simulink model "demo_FIXS"  (R2024a)
settings: Solver=VariableStepAuto  StartTime=0.0  StopTime=10.0  RelTol=1e-3
PostLoadFcn:
  | if any(exist('dsrtsu_mdlpostloadfcn', 'file') ~= 0), dsrtsu_mdlpostloadfcn('Execute', bdroot); end
InitFcn:
  | , if any(exist('dsmpb_private', 'file') ~= 0), dsmpb_private('dsmpb_mdlclblib', 'Init', bdroot); end,
values from neighbouring files (symbols this model uses):
  RealSimPara =     [Run_Simulink.mat]
libraries: dsmpblib x7, simulink x2
PreSaveFcn:
  | , if any(exist('dsmpb_private', 'file') ~= 0), dsmpb_private('dsmpb_mdlclblib', 'PreSave', bdroot); end,
CloseFcn:
  | , if any(exist('dsmpb_private', 'file') ~= 0), dsmpb_private('dsmpb_mdlclblib', 'Close', bdroot); end,
settings Model: DSMPB_ID_DATA={'114',struct('BlockId','a362e819-36dc-4974-aa36-3021815529a3','SignalIds',{{'66e99ec9-adbb-4575-a499-7c125ba92483'}}),'126',struct('BlockId','ae842df5-44fe-466f-9c27-a215b2028e86','SignalIds',{{'c9fc9f6b-9f86-4efb-bbc4-57bab20bb633'}}),'127',struct('BlockId','bbe675d0-07e1-4678-85bf-fdbba0576f1e','SignalIds',{{'fbad8ef8-ed8e-4d52-83c5-289887b658bf','bfa4259a-ff07-4a65-a7c9-9af4643f0ea5','da3d735e-2e4d-4dbe-9156-097bd40e1eb5','0aaec2e5-1bc6-40e3-804f-bcf62d1171e8'}}),'128',struct('BlockId','76c42765-af6a-43b1-a646-d573c8b7c57f','SignalIds',{{'afa686ea-bff9-4ae8-bbc4-1f85da76ddbd'}}),'129',struct('BlockId','547cde89-fa54-43bb-91af-f85d56e956d9','SignalIds',{{'71dcf01e-4040-4f0f-9727-35b21fbf9010'}}),'134',struct('BlockId','2d3928d4-db37-4811-a604-a01aef7cb2d7','SignalIds',{{'b231ed0e-9922-4662-b18e-0578afdeacb1','d97ae3f2-e654-4125-b1b8-791beb64344e'}}),'147',struct('BlockId','e4d38646-31b4-470f-bd5f-0342a996991a','SignalIds',{{'19e5aa06-a56a-40dc-84e8-1ac500eeaf07','77e1adf7-a3b1-4325-a85b-daf2ff9418b5','6e5fcfab-5f3b-494e-8d3b-0a2c9e0cd453'}})}  Creator=MSC_Lab  LastModifiedBy=MSC_Lab

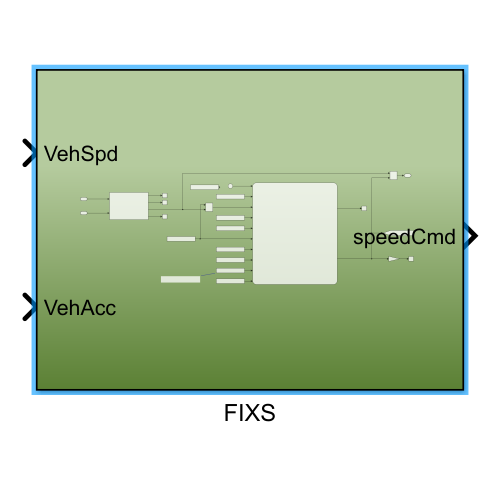
[thumbnail: Simulink's stored preview of the top-level diagram]
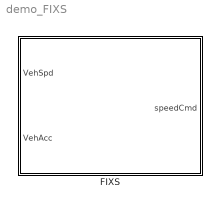
== system demo_FIXS ==
  FIXS : Subsystem

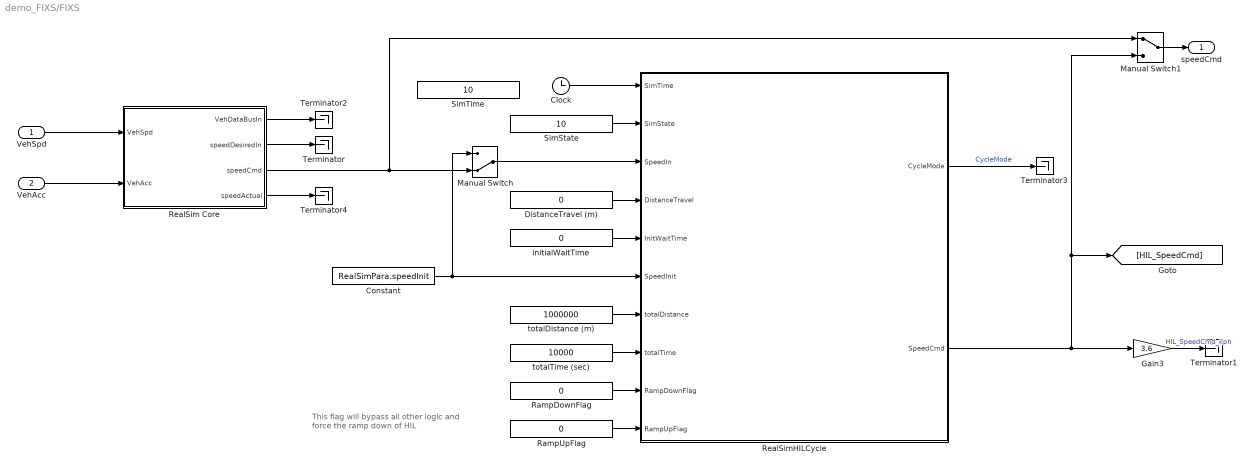
== system demo_FIXS/FIXS ==
  note: This flag will bypass all other logic and force the ramp down of HIL
  VehSpd : Inport
  VehAcc : Inport  Port=2
  Clock : Clock
  Constant : Constant  Value=RealSimPara.speedInit
  DistanceTravel (m) : Constant  Value=0
  Gain3 : Gain  Gain=3.6
  Manual Switch : ManualSwitch  CurrentSetting=0
  Manual Switch1 : ManualSwitch
  RampDownFlag : Constant  Value=0
  RampUpFlag : Constant  Value=0
  RealSim Core : Subsystem
  RealSimHILCycle : Stateflow chart  TreatAsAtomicUnit=on
  SimState : Constant  Value=10
  SimTime : Constant  Value=10
  Terminator{,1..4} (5 alike) : Terminator
  initialWaitTime : Constant  Value=0
  totalDistance (m) : Constant  Value=1000000
  totalTime (sec) : Constant  Value=10000
  speedCmd : Outport
  wires:
  RealSim Core/2(speedDesiredIn) -> Terminator/1
  RampDownFlag/1 -> RealSimHILCycle/9(RampDownFlag)
  totalDistance (m)/1 -> RealSimHILCycle/7(totalDistance)
  Manual Switch/1 -> RealSimHILCycle/3(SpeedIn)
  Gain3/1 -> Terminator1/1  "HIL_SpeedCmd_kph"
  totalTime (sec)/1 -> RealSimHILCycle/8(totalTime)
  RealSimHILCycle/1(CycleMode) -> Terminator3/1  "CycleMode"
  initialWaitTime/1 -> RealSimHILCycle/5(InitWaitTime)
  RealSimHILCycle/2(SpeedCmd) -> [HIL_SpeedCmd], Manual Switch1/2, Gain3/1
  Constant/1 -> Manual Switch/1, RealSimHILCycle/6(SpeedInit)
  Manual Switch1/1 -> speedCmd/1
  RealSim Core/3(speedCmd) -> Manual Switch1/1, Manual Switch/2
  RampUpFlag/1 -> RealSimHILCycle/10(RampUpFlag)
  VehSpd/1 -> RealSim Core/1(VehSpd)
  RealSim Core/1(VehDataBusIn) -> Terminator2/1
  RealSim Core/4(speedActual) -> Terminator4/1
  DistanceTravel (m)/1 -> RealSimHILCycle/4(DistanceTravel)
  SimState/1 -> RealSimHILCycle/2(SimState)
  Clock/1 -> RealSimHILCycle/1(SimTime)
  VehAcc/1 -> RealSim Core/2(VehAcc)

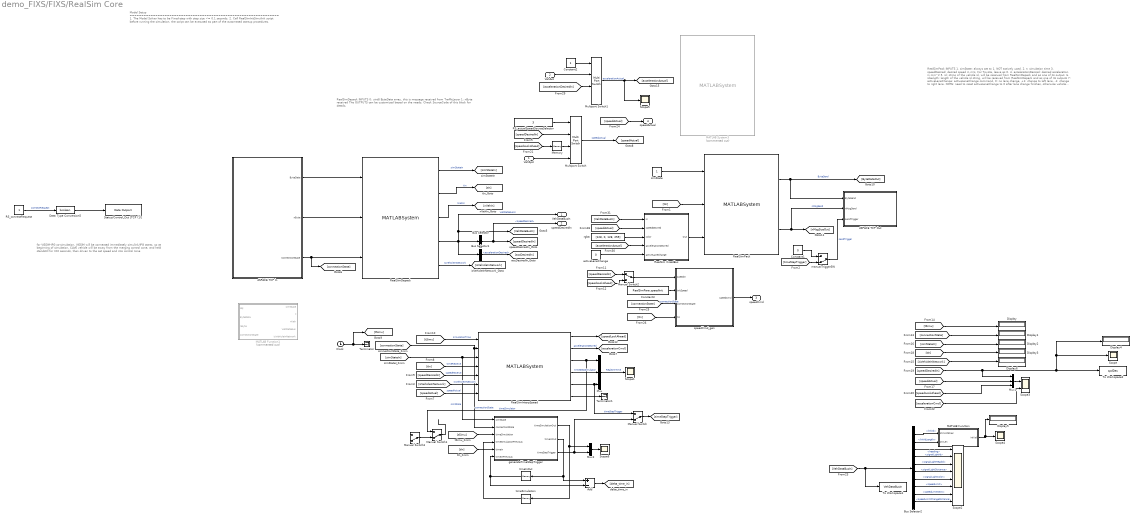
== system demo_FIXS/FIXS/RealSim Core ==
  note: Model Setup
      | ================================================================
      | 1. The Model Solver has to be Fixed-step with step size <= 0.1 seconds.
      | 2. Call RealSimInitSimulink script before running the simulation. the script can be executed as part of the automated startup procedures.
  note: RealSimDepack
      | INPUTS
      | 0: uint8 ByteData array, this is message received from TrafficLayer
      | 1: nByte received
      |
      | The OUTPUTS can be customized based on the needs. Check SourceCode of this block for details.
  note: RealSimPack
      | INPUTS
      | 1. simState: always set to 1. NOT actively used.
      | 2. t: simulation time
      | 3. speedDesired: desired speed in m/s, For Toyota, leave as 0.
      | 4. accelerationDesired: desired acceleration in m/s^2
      | 5. id: string of the vehicle id, will be received from RealSimDepack and as one of its output.
      | 6. idLength: length of the vehicle id string, will be received from RealSimDepack and as one of its outputs
      | 7: activeLaneChange: activeLaneChange command, 0: no lane change, +1: change to left lane, -1: change to right lane. NOTE: need to reset activeLaneChange to 0 after lane change finishes, otherwise vehicle will keep making lane change. Will receive 0 activeLaneChangeFdbk from RealSimDepack when lane change finishes.
      |
      | NOTE 1: Currently, only speedDesired and/or accelerationDesired can be sent to VISSIM/SUMO. The data format receive and send are the same so other mesage fields of the send data are irrelevant and can be set to empty or zero.
      |
      | NOTE 2: if select both speedDesired and accelerationDesired
      | in config.yaml, then only accelerationDesired will be used
      | to control vehicles in TrafficSimulator. if only one of
      | speedDesired and accelerationDesired selected in
      | config.yaml, then the one selected will be used for
      | control, the other input can be leave as 0.
      |
      | NOTE 3: for VISSIM, speedDesired or accelerationDesired will be the control command 0.2 seconds in the future.
      |
      | OUTPUTS
      | 1.ByteData: bytes vector that will be sent to TrafficSimualtor
      | 2.nMsgSize: size of bytes to be sent
  note: for VISSIM-IPG co-simulation, VISSIM will be connected immediately simulink/IPG starts. so at beginning of simulation, CAVE vehicle will be away from the merging control zone, and held standstill for XXX seconds, then driven to the set speed and into control zone
  VehSpd : Inport
  VehAcc : Inport  Port=2
  Add : Sum  Inputs=+-
  Bus Selector : BusSelector  OutputSignals=speedDesired
  Bus Selector1 : BusSelector  OutputSignals=accelerationDesired
  Bus Selector2 : BusSelector  OutputSignals=linkId,linkIdLength,heading,signalLightId,signalLightHeadId,signalLightDistance,signalLightColor,speedLimit,speedLimitNext,speedLimitChangeDistance
  Clock : Clock
  Constant1 : Constant  Value=0
  Constant2 : Constant
  Constant3 : Constant  Value=RealSimPara.speedInit
  Data Type Conversion5 : DataTypeConversion  OutDataTypeStr=boolean  SaturateOnIntegerOverflow=off  RndMeth=Floor
  Display{,1..6} (7 alike) : Display
  MATLAB Function : MATLAB Function  TreatAsAtomicUnit=on
  MATLAB Function1 : MATLAB Function  Commented=on  TreatAsAtomicUnit=on
  MATLAB System3 : MATLABSystem  Commented=on  System=RealSimPack  VehicleMessageFieldDefInputVec=VehicleMessageFieldDefInputVec  SimulateUsing=Code generation
      mask Type: RealSimPack
      mask Display:
      | disp('RealSimPack');
      | port_label('input',1,'simState');
      | port_label('input',2,'t');
      | port_label('input',3,'VehDataBus');
      | port_label('output',1,'ByteData');
      | port_label('output',2,'nMsgSize');
  Manual Switch : ManualSwitch  CurrentSetting=0
  Manual Switch1 : ManualSwitch  CurrentSetting=0
  Manual Switch2 : ManualSwitch
  Manual Switch3 : ManualSwitch  CurrentSetting=0
  Memory : Memory
  Multiport Switch : MultiPortSwitch  SaturateOnIntegerOverflow=off  InputSameDT=off
  Multiport Switch1 : MultiPortSwitch  SaturateOnIntegerOverflow=off  InputSameDT=off
  Mux : Mux  Inputs=3
  Mux1 : Mux  Inputs=3
  Mux2 : Mux  Inputs=2
  RS_actualSpeedSourceSelector : Constant  Value=3
  RS_connectRequest : Constant
  RealSim CreatBus : Subsystem
  RealSimDepack : MATLABSystem  System=RealSimDepack  OutputBusName=VehDataBus  VehicleMessageFieldDefInputVec=VehicleMessageFieldDefInputVec  SimulateUsing=Code generation
      mask Type: RealSimDepack
      mask Display:
      | disp('RealSimDepack');
      | port_label('input',1,'ByteData');
      | port_label('input',2,'nByte');
      | port_label('input',3,'connectionState');
      | port_label('output',1,'simState');
      | port_label('output',2,'t');
      | port_label('output',3,'nVeh');
      | port_label('output',4,'VehDataBus');
      | port_label('output',5,'isVehicleInNetwork');
  RealSimInterpSpeed : MATLABSystem  System=RealSimInterpSpeed  initialSpeed=RealSimPara.speedInit  speedLookAheadHorizon=RealSimPara.tLookahead  speedUpperBound=30  smoothWindow=RealSimPara.smoothWindow  SimulateUsing=Code generation
      mask Type: RealSimInterpSpeed
      mask Display:
      | disp('RealSimInterpSpeed');
      | port_label('input',1,'simulationTime');
      | port_label('input',2,'connectionState');
      | port_label('input',3,'simState');
      | port_label('input',4,'timeReceive');
      | port_label('input',5,'speedReceive');
      | port_label('input',6,'isVehicleInNetwork');
      | port_label('input',7,'speedActual');
      | port_label('output',1,'speedLookAhead');
      | port_label('output',2,'accelerationDesired');
      | port_label('output',3,'timeSimulator');
      | port_label('output',4,'timeStepSimulator');
      | port_label('output',5,'timeStepTrigger');
      | port_label('output',6,'RealSimDelay');
  RealSimPack : MATLABSystem  System=RealSimPack  VehicleMessageFieldDefInputVec=VehicleMessageFieldDefInputVec  SimulateUsing=Code generation
      mask Type: RealSimPack
      mask Display:
      | disp('RealSimPack');
      | port_label('input',1,'simState');
      | port_label('input',2,'t');
      | port_label('input',3,'VehDataBus');
      | port_label('output',1,'ByteData');
      | port_label('output',2,'nMsgSize');
  Scope{,1,4..6} (5 alike) : Scope
  Scope2 : Scope  NumInputPorts=8
  Scope3 : Scope  NumInputPorts=2
  Status/Control_Out [TCP (1)] : dsmpblib/Data Outport  Priority=-10000
      settings: SourceProductName=dSPACE Model Interface Package for Simulink (MIPS)
  Terminator : Terminator
  Terminator1 : Terminator
  To Workspace1 : ToWorkspace  VariableName=VehDataBusIn  SaveFormat=Timeseries  SampleTime=-1
  To Workspace2 : ToWorkspace  VariableName=spdDes  SaveFormat=Structure With Time  SampleTime=-1
  activeLaneChange : Constant  Value=0
  dSPACE TCP In : Subsystem
  dSPACE TCP Out : Subsystem
  generateTimeStepTrigger : MATLAB Function  TreatAsAtomicUnit=on
  manualTriggerSW : ManualSwitch  CurrentSetting=0
  rgba : Constant  Value=[128, 0, 128, 255]
  simState : Constant
  speedCmd_gen : Subsystem
  timeInOut : Memory
  timeSimulation : Memory
  VehDataBusIn : Outport
  speedDesiredIn : Outport  Port=2
  speedCmd : Outport  Port=3
  speedActual : Outport  Port=4
  wires:
  [speedLookAhead] -> Memory/1
  Bus Selector/1 -> speedDesiredIn/1, [speedDesiredIn]  "<speedDesired>"
  RealSimDepack/1 -> [simStateIn]  "simStateIn"
  Bus Selector2/9 -> Scope2/7  "<speedLimitNext>"
  [tSimu] -> RealSimInterpSpeed/1  "simulationTime"
  RealSimInterpSpeed/4 -> Mux/2  "timeStepSimulator"
  Bus Selector2/1 -> MATLAB Function/1(strUint8Vec)  "<linkId>"
  Bus Selector2/3 -> Scope2/1  "<heading>"
  [tIn] -> RealSimInterpSpeed/4  "timeReceive"
  Bus Selector2/10 -> Scope2/8  "<speedLimitChangeDistance>"
  VehSpd/1 -> Multiport Switch/4
  [speedDesiredIn] -> RealSimInterpSpeed/5  "speedReceive"
  [simStateIn] -> Display2/1
  RealSimDepack/3 -> [nVehIn]  "nVehIn"
  [VehDataBusIn] -> To Workspace1/1, Bus Selector2/1
  [isVehicleInNetwork] -> Display6/1
  Bus Selector2/7 -> Scope2/5  "<signalLightColor>"
  simState/1 -> RealSimPack/1
  RealSimDepack/4 -> Bus Selector1/1, VehDataBusIn/1, [VehDataBusIn], Bus Selector/1  "VehDataBusIn"
  [speedDesiredIn] -> Display4/1, Scope/1, To Workspace2/1, Mux1/1
  RealSimInterpSpeed/2 -> [accelerationCmd]  "accelerationDesired"
  [isVehicleInNetwork] -> RealSimInterpSpeed/6  "isVehicleInNetwork"
  RS_actualSpeedSourceSelector/1 -> Multiport Switch/1
  RealSim CreatBus/1(Out) -> RealSimPack/3
  [accelerationCmd] -> Scope3/2
  Mux/1 -> Scope1/1  "RealSimTime"
  [tIn] -> RealSimPack/2
  Bus Selector2/2 -> MATLAB Function/2(strLen)  "<linkIdLength>"
  Bus Selector2/8 -> Scope2/6  "<speedLimit>"
  [connectionState] -> Display1/1
  RealSimInterpSpeed/5 -> Manual Switch/1, Mux/3  "timeStepTrigger"
  RealSimDepack/5 -> [isVehicleInNetwork]  "isVehicleInNetwork"
  Bus Selector2/5 -> Scope2/3  "<signalLightHeadId>"
  Bus Selector2/6 -> Scope2/4  "<signalLightDistance>"
  RealSimInterpSpeed/6 -> Terminator1/1
  RealSimPack/1 -> dSPACE TCP Out/1(ByteSend), [ByteDataOut]  "ByteSend"
  [tIn] -> Display3/1
  Multiport Switch/1 -> [speedActual]  "speedActual"
  [tSimu] -> Display/1
  [connectionState] -> generateTimeStepTrigger/2(connectionState), RealSimInterpSpeed/2  "connectionState"
  [speedLookAhead] -> Mux1/3
  [speedActual] -> RealSimInterpSpeed/7  "speedActual"
  [simStateIn] -> generateTimeStepTrigger/1(simState), RealSimInterpSpeed/3  "simState"
  RealSimInterpSpeed/1 -> [speedLookAhead]
  Mux1/1 -> Scope3/1
  MATLAB Function/1(intVal) -> Display5/1, Scope4/1
  RealSimPack/2 -> dSPACE TCP Out/2(nMsgSend), [nMsgSizeOut]  "nMsgSend"
  Bus Selector2/4 -> Scope2/2  "<signalLightId>"
  RealSimInterpSpeed/3 -> Mux/1, Manual Switch1/1  "timeSimulator"
  [speedDesiredIn] -> Multiport Switch/2
  [speedActual] -> Mux1/2
  RealSimDepack/2 -> [tIn]  "tIn"
  manualTriggerSW/1 -> dSPACE TCP Out/3(sendTrigger)  "sendTrigger"
  dSPACE TCP In/3(ConnectionState) -> RealSimDepack/3, [connectionState]
  dSPACE TCP In/1(ByteData) -> RealSimDepack/1
  dSPACE TCP In/2(nByte) -> RealSimDepack/2
  Data Type Conversion5/1 -> Status/Control_Out [TCP (1)]/1
  RS_connectRequest/1 -> Data Type Conversion5/1  "connectRequest"
  Memory/1 -> Multiport Switch/3
  Clock/1 -> Terminator/1, [tSimu]
  timeSimulation/1 -> generateTimeStepTrigger/4(timeSimulationPrevious)
  generateTimeStepTrigger/3(timeStepTrigger) -> Manual Switch/2, Mux2/2
  generateTimeStepTrigger/1(timeSimulationOut) -> Mux2/1, timeSimulation/1
  Mux2/1 -> Scope6/1
  Manual Switch/1 -> [timeStepTrigger]
  [timeStepTrigger] -> manualTriggerSW/2
  Constant1/1 -> manualTriggerSW/1
  ? -> Manual Switch3/1
  [speedDesiredIn] -> Manual Switch2/1
  [speedLookAhead] -> Manual Switch2/2
  [speedActual] -> speedActual/1
  Manual Switch2/1 -> speedCmd_gen/1(speedIn)
  Constant3/1 -> speedCmd_gen/2(initSpeed)
  speedCmd_gen/1(speedCmd) -> speedCmd/1
  [connectionState] -> speedCmd_gen/3(connectionState)  "connectionState"
  [tIn] -> speedCmd_gen/4(tIn)
  ? -> Manual Switch3/2
  Manual Switch3/1 -> Manual Switch1/2
  generateTimeStepTrigger/2(timeInOut) -> Add/1, timeInOut/1
  timeInOut/1 -> Add/2, generateTimeStepTrigger/6(timeInPrevious)
  [VehDataBusIn] -> RealSim CreatBus/1(In)
  rgba/1 -> RealSim CreatBus/3(color)
  activeLaneChange/1 -> RealSim CreatBus/5(activeLaneChange)
  [speedActual] -> RealSim CreatBus/2(speedDesired)
  Bus Selector1/1 -> [accDesiredIn]  "<accelerationDesired>"
  [accelerationDesiredIn] -> Multiport Switch1/3
  VehAcc/1 -> Multiport Switch1/2
  Constant2/1 -> Multiport Switch1/1
  Multiport Switch1/1 -> [accelerationActual], Scope5/1  "accelerationActual"
  [accelerationActual] -> RealSim CreatBus/4(accelerationDesired)
  Manual Switch1/1 -> ?
  [tSimu] -> generateTimeStepTrigger/3(timeSimulation)
  [tIn] -> generateTimeStepTrigger/5(timeIn)
  Add/1 -> [delta_time_in]

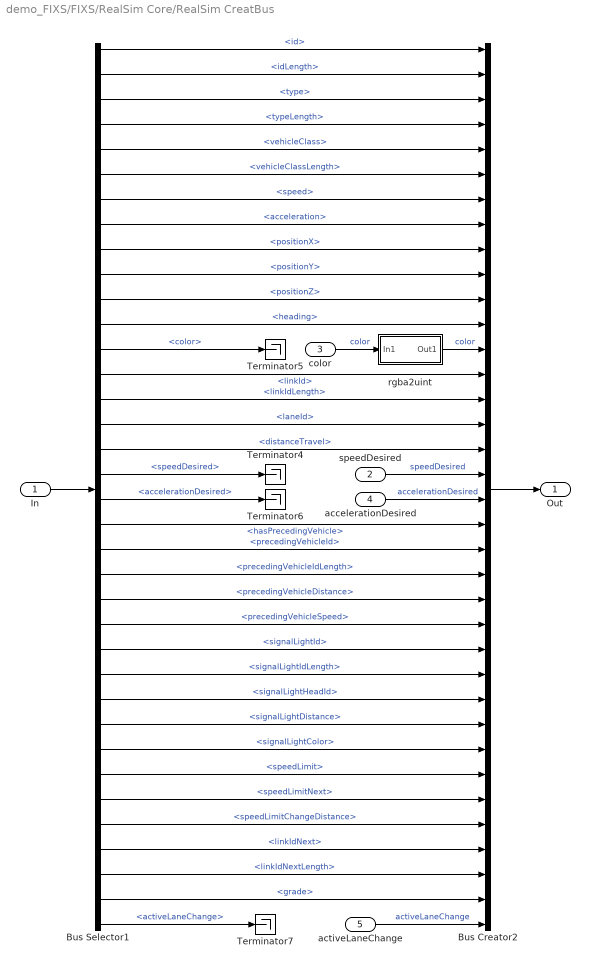
== system demo_FIXS/FIXS/RealSim Core/RealSim CreatBus ==
  In : Inport
  speedDesired : Inport  Port=2
  color : Inport  Port=3
  accelerationDesired : Inport  Port=4
  activeLaneChange : Inport  Port=5
  Bus Creator2 : BusCreator  Inputs=36  OutDataTypeStr=Bus: VehDataBus
  Bus Selector1 : BusSelector  OutputSignals=id,idLength,type,typeLength,vehicleClass,vehicleClassLength,speed,acceleration,positionX,positionY,positionZ,heading,color,linkId,linkIdLength,laneId,distanceTravel,speedDesired,accelerationDesired,hasPrecedingVehicle,precedingVehicleId,precedingVehicleIdLength,precedingVehicleDistance,precedingVehicleSpeed,signalLightId,signalLightIdLength,signalLightHeadId,signalLightDistance,signalLightColor,speedLimit,speedLimitNext,speedLimitChangeDistance,linkIdNext,linkIdNextLength,grade,activeLaneChange
  Terminator{4..7} (4 alike) : Terminator
  rgba2uint : Subsystem
  Out : Outport
  wires:
  Bus Creator2/1 -> Out/1
  rgba2uint/1(Out1) -> Bus Creator2/13  "color"
  color/1 -> rgba2uint/1(In1)  "color"
  accelerationDesired/1 -> Bus Creator2/19  "accelerationDesired"
  speedDesired/1 -> Bus Creator2/18  "speedDesired"
  activeLaneChange/1 -> Bus Creator2/36  "activeLaneChange"
  Bus Selector1/36 -> Terminator7/1  "<activeLaneChange>"
  Bus Selector1/35 -> Bus Creator2/35  "<grade>"
  Bus Selector1/34 -> Bus Creator2/34  "<linkIdNextLength>"
  Bus Selector1/33 -> Bus Creator2/33  "<linkIdNext>"
  Bus Selector1/32 -> Bus Creator2/32  "<speedLimitChangeDistance>"
  Bus Selector1/31 -> Bus Creator2/31  "<speedLimitNext>"
  Bus Selector1/30 -> Bus Creator2/30  "<speedLimit>"
  Bus Selector1/29 -> Bus Creator2/29  "<signalLightColor>"
  Bus Selector1/28 -> Bus Creator2/28  "<signalLightDistance>"
  Bus Selector1/27 -> Bus Creator2/27  "<signalLightHeadId>"
  Bus Selector1/26 -> Bus Creator2/26  "<signalLightIdLength>"
  Bus Selector1/25 -> Bus Creator2/25  "<signalLightId>"
  Bus Selector1/24 -> Bus Creator2/24  "<precedingVehicleSpeed>"
  Bus Selector1/23 -> Bus Creator2/23  "<precedingVehicleDistance>"
  Bus Selector1/22 -> Bus Creator2/22  "<precedingVehicleIdLength>"
  Bus Selector1/21 -> Bus Creator2/21  "<precedingVehicleId>"
  Bus Selector1/20 -> Bus Creator2/20  "<hasPrecedingVehicle>"
  Bus Selector1/19 -> Terminator6/1  "<accelerationDesired>"
  Bus Selector1/18 -> Terminator4/1  "<speedDesired>"
  Bus Selector1/17 -> Bus Creator2/17  "<distanceTravel>"
  Bus Selector1/16 -> Bus Creator2/16  "<laneId>"
  Bus Selector1/15 -> Bus Creator2/15  "<linkIdLength>"
  Bus Selector1/14 -> Bus Creator2/14  "<linkId>"
  Bus Selector1/13 -> Terminator5/1  "<color>"
  Bus Selector1/12 -> Bus Creator2/12  "<heading>"
  Bus Selector1/11 -> Bus Creator2/11  "<positionZ>"
  Bus Selector1/10 -> Bus Creator2/10  "<positionY>"
  Bus Selector1/9 -> Bus Creator2/9  "<positionX>"
  Bus Selector1/8 -> Bus Creator2/8  "<acceleration>"
  Bus Selector1/7 -> Bus Creator2/7  "<speed>"
  Bus Selector1/6 -> Bus Creator2/6  "<vehicleClassLength>"
  Bus Selector1/5 -> Bus Creator2/5  "<vehicleClass>"
  Bus Selector1/4 -> Bus Creator2/4  "<typeLength>"
  Bus Selector1/3 -> Bus Creator2/3  "<type>"
  Bus Selector1/2 -> Bus Creator2/2  "<idLength>"
  Bus Selector1/1 -> Bus Creator2/1  "<id>"
  In/1 -> Bus Selector1/1

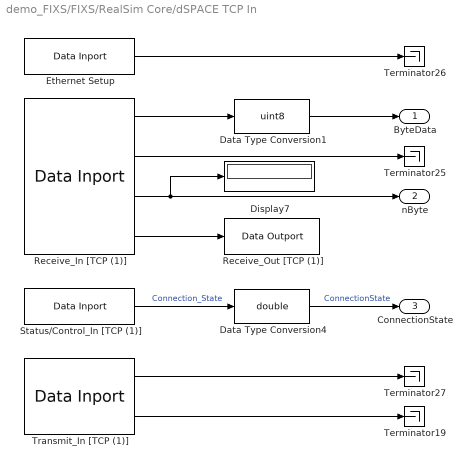
== system demo_FIXS/FIXS/RealSim Core/dSPACE TCP In ==
  Data Type Conversion1 : DataTypeConversion  OutDataTypeStr=uint8  SaturateOnIntegerOverflow=off  RndMeth=Floor
  Data Type Conversion4 : DataTypeConversion  OutDataTypeStr=double  SaturateOnIntegerOverflow=off  RndMeth=Floor
  Display7 : Display
  Ethernet Setup : dsmpblib/Data Inport  Priority=10000
      settings: SourceProductName=dSPACE Model Interface Package for Simulink (MIPS)
  Receive_In [TCP (1)] : dsmpblib/Data Inport  Priority=10000
      settings: SourceProductName=dSPACE Model Interface Package for Simulink (MIPS)
  Receive_Out [TCP (1)] : dsmpblib/Data Outport  Priority=-10000
      settings: SourceProductName=dSPACE Model Interface Package for Simulink (MIPS)
  Status/Control_In [TCP (1)] : dsmpblib/Data Inport  Priority=10000
      settings: SourceProductName=dSPACE Model Interface Package for Simulink (MIPS)
  Terminator{19,25..27} (4 alike) : Terminator
  Transmit_In [TCP (1)] : dsmpblib/Data Inport  Priority=10000
      settings: SourceProductName=dSPACE Model Interface Package for Simulink (MIPS)
  ByteData : Outport
  nByte : Outport  Port=2
  ConnectionState : Outport  Port=3
  wires:
  Data Type Conversion4/1 -> ConnectionState/1  "ConnectionState"
  Status/Control_In [TCP (1)]/1 -> Data Type Conversion4/1  "Connection_State"
  Receive_In [TCP (1)]/4 -> Receive_Out [TCP (1)]/1
  Ethernet Setup/1 -> Terminator26/1
  Receive_In [TCP (1)]/1 -> Data Type Conversion1/1
  Transmit_In [TCP (1)]/2 -> Terminator19/1
  Transmit_In [TCP (1)]/1 -> Terminator27/1
  Receive_In [TCP (1)]/2 -> Terminator25/1
  Receive_In [TCP (1)]/3 -> nByte/1, Display7/1
  Data Type Conversion1/1 -> ByteData/1

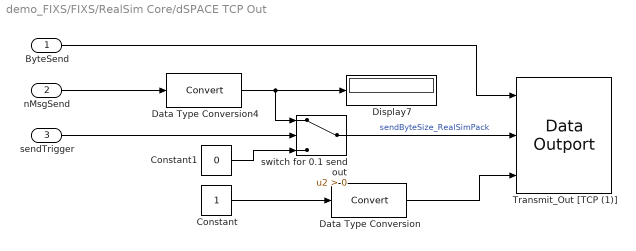
== system demo_FIXS/FIXS/RealSim Core/dSPACE TCP Out ==
  ByteSend : Inport
  nMsgSend : Inport  Port=2
  sendTrigger : Inport  Port=3
  Constant : Constant
  Constant1 : Constant  Value=0
  Data Type Conversion : DataTypeConversion  SaturateOnIntegerOverflow=off  RndMeth=Floor
  Data Type Conversion4 : DataTypeConversion  SaturateOnIntegerOverflow=off  RndMeth=Floor
  Display7 : Display
  Transmit_Out [TCP (1)] : dsmpblib/Data Outport  Priority=-10000
      settings: SourceProductName=dSPACE Model Interface Package for Simulink (MIPS)
  switch for 0.1 send out : Switch  Criteria=u2 > Threshold  SaturateOnIntegerOverflow=off  InputSameDT=off
  wires:
  Constant1/1 -> switch for 0.1 send out/3
  nMsgSend/1 -> Data Type Conversion4/1
  Data Type Conversion4/1 -> switch for 0.1 send out/1, Display7/1
  switch for 0.1 send out/1 -> Transmit_Out [TCP (1)]/2  "sendByteSize_RealSimPack"
  sendTrigger/1 -> switch for 0.1 send out/2
  Constant/1 -> Data Type Conversion/1
  Data Type Conversion/1 -> Transmit_Out [TCP (1)]/3
  ByteSend/1 -> Transmit_Out [TCP (1)]/1

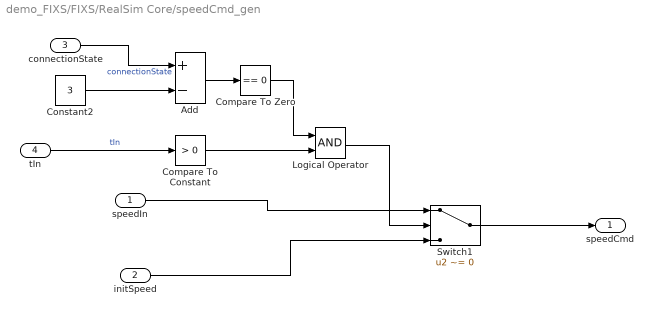
== system demo_FIXS/FIXS/RealSim Core/speedCmd_gen ==
  speedIn : Inport
  initSpeed : Inport  Port=2
  connectionState : Inport  Port=3
  tIn : Inport  Port=4
  Add : Sum  Inputs=+-
  Compare To Constant : simulink/Logic and Bit Operations/Compare To Constant  relop=>  const=0  OutDataTypeStr=boolean
  Compare To Zero : simulink/Logic and Bit Operations/Compare To Zero  relop===  OutDataTypeStr=boolean
  Constant2 : Constant  Value=3
  Logical Operator : Logic  AllPortsSameDT=off  OutDataTypeStr=boolean
  Switch1 : Switch  Criteria=u2 ~= 0  SaturateOnIntegerOverflow=off  InputSameDT=off
  speedCmd : Outport
  wires:
  Add/1 -> Compare To Zero/1
  initSpeed/1 -> Switch1/3
  Constant2/1 -> Add/2
  Switch1/1 -> speedCmd/1
  connectionState/1 -> Add/1  "connectionState"
  speedIn/1 -> Switch1/1
  tIn/1 -> Compare To Constant/1  "tIn"
  Compare To Constant/1 -> Logical Operator/2
  Logical Operator/1 -> Switch1/2
  Compare To Zero/1 -> Logical Operator/1

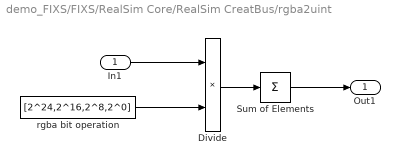
== system demo_FIXS/FIXS/RealSim Core/RealSim CreatBus/rgba2uint ==
  In1 : Inport
  Divide : Product  Inputs=**
  Sum of Elements : Sum  Inputs=+
  rgba bit operation : Constant  Value=[2^24,2^16,2^8,2^0]
  Out1 : Outport
  wires:
  Sum of Elements/1 -> Out1/1
  rgba bit operation/1 -> Divide/2
  In1/1 -> Divide/1
  Divide/1 -> Sum of Elements/1

== stateflow chart demo_FIXS/FIXS/RealSimHILCycle ==
  state CycleOn
    state InitialWait
      CycleMode=1;
    state RampUp
      CycleMode=2;
      SpeedCmd=SpeedCmd+0.1
    state Driving
      CycleMode=3;
      SpeedCmd=max(SpeedIn, 0)
    state WaitForNextRamp
    InitialWait -> RampUp : [after(InitWaitTime,sec) || RampUpFlag]
    (default) -> InitialWait
    RampUp -> Driving [order 1] : [abs(SpeedCmd-SpeedInit)<0.5 && abs(SpeedCmd)>0 ]
    RampUp -> CycleOn.WaitForNextRamp [order 2] : [abs(SpeedCmd-SpeedInit)>=0.1]
    CycleOn.WaitForNextRamp -> RampUp : after(0.1,sec)
  state Idle
    CycleMode=0;
    SpeedCmd=0;
    CycleTime=0;
  state RampDown
    CycleMode=4;
    SpeedCmd=SpeedCmd-1;
  state WaitForNextRamp
  (default) -> Idle
  Idle -> CycleOn : [SimState>=6 && ...
      | DistanceTravel <= totalDistance && ...
      | SimTime <= totalTime && ...
      | ~RampDownFlag]
  RampDown -> Idle [order 1] : [SpeedCmd<0.5]
  CycleOn -> RampDown : [DistanceTravel > totalDistance || ...
      | SimTime > totalTime || ...
      | RampDownFlag || ...
      | SimState==9]
  WaitForNextRamp -> RampDown : after(0.1,sec)
  RampDown -> WaitForNextRamp [order 2] : [SpeedCmd>=0.5]
  data: SimTime input; SimState input; SpeedIn input; DistanceTravel input; InitWaitTime input; SpeedInit input; totalDistance input; CycleMode output; SpeedCmd output; totalTime input; RampDownFlag input; CycleTime local; RampUpFlag input

== matlab function demo_FIXS/FIXS/RealSim Core/MATLAB Function ==
  data: strUint8Vec input; intVal output double; strLen input
function intVal = strVec2Int(strUint8Vec, strLen)

    strVec = blanks(50);
    for i = 1:strLen
       strVec(i) = strUint8Vec(i); 
    end
    if strLen > 0
        intVal = real(str2double(strVec(1:strLen)));
    else
        intVal = -1;
    end

== matlab function demo_FIXS/FIXS/RealSim Core/MATLAB Function1 ==
  data: obj input; simState output; ByteData input; nByte input; connectionState input; t output; nVeh output; VehDataBus output; isVehicleInNetwork output
function [simState, t, nVeh, VehDataBus, isVehicleInNetwork] = stepImpl(obj, ByteData, nByte, connectionState)

    simState = obj.simStatePrevious;
    t = obj.tPrevious;
    nVeh = 0;
    
    % init values for other variables
    totalMsgSize = 0; % this is the total message size received from Real-Sim
    msgProcessed = 0; % to record how many messages have been processed
    
    VehDataBus = obj.VehicleDataPrevious;

    %---------------------------
    % read received buffer
    %---------------------------
    % need to check size, before connection, there could be no
    % message at all             
    if nByte >= obj.msgHeaderSize
        simState = double(typecast(uint8(ByteData(1)),'uint8'));
        t = double(typecast(uint8(ByteData(2:5)),'single'));
        totalMsgSize = double(typecast(uint8(ByteData(6:9)),'uint32'));
        msgProcessed = obj.msgHeaderSize;
        
        obj.simStatePrevious = simState;
        obj.tPrevious = t;
    end
    
    % read actual message fields
    while round(msgProcessed) < round(totalMsgSize)
        iMsgSizeRecv = double(typecast(uint8(ByteData(msgProcessed+1:msgProcessed+2)),'uint16'));
        iMsgTypeRecv = double(typecast(uint8(ByteData(msgProcessed+3)),'uint8'));

        % !!! for now, Simulink only supports vehicle data type
        if obj.enableDebug
            obj.vehMsgIdentifer = iMsgTypeRecv;
        else
            obj.vehMsgIdentifer = 1;
        end
        
        if iMsgTypeRecv == obj.vehMsgIdentifer
            VehDataBus = obj.depackVehData(VehDataBus, ByteData(msgProcessed+obj.msgEachHeaderSize+1:msgProcessed+iMsgSizeRecv));
               
            nVeh = nVeh + 1;

            obj.VehicleDataPrevious = VehDataBus;
            obj.isVehicleInNetworkPrevious = 1;
        else
            % not supported yet!!!
            
        end
        
        msgProcessed = msgProcessed + iMsgSizeRecv;

    end
    

    if abs(connectionState-3)>1e-5
        % if not connected, then set to 0
        obj.simStatePrevious = 0;
        obj.tPrevious = 0;
        obj.nVehPrevious = 0;
        obj.VehicleDataPrevious = obj.VehicleDataEmpty;
        obj.isVehicleInNetworkPrevious = 0;
    else
        if totalMsgSize == 9
            obj.isVehicleInNetworkPrevious = 0;
        end
    end
    isVehicleInNetwork = obj.isVehicleInNetworkPrevious;

== matlab function demo_FIXS/FIXS/RealSim Core/generateTimeStepTrigger ==
  data: simState input; connectionState input; timeSimulation input; timeSimulationOut output; timeInOut output; timeSimulationPrevious input; timeStepTrigger output; timeIn input; timeInPrevious input
function [timeSimulationOut, timeInOut, timeStepTrigger]  = fcn(simState, connectionState, timeSimulation, timeSimulationPrevious, timeIn, timeInPrevious)


%if simState && abs(connectionState-3) < 1e-5 && (timeSimulator >= timeStepSimulatorPrevious + 0.1 - 1e-5 || abs(timeSimulator) < 1e-5)
% if simState && abs(connectionState-3) < 1e-5 && (timeSimulation >= timeSimulationPrevious + 0.1 - 1e-5)
if simState && abs(connectionState-3) < 1e-5 && ((timeSimulation >= timeSimulationPrevious + 0.1 - 1e-5) && (timeIn >= timeInPrevious + 0.1 - 1e-3))
    timeSimulationOut = timeSimulation;
    timeInOut = timeIn;
    timeStepTrigger = 1;
else
    timeSimulationOut = timeSimulationPrevious;
    timeInOut = timeInPrevious;
    timeStepTrigger = 0;
end
